simulink model "PMSM_STATE_SS_AR222"  (R2021a)
settings: Solver=ode45  StartTime=0.0  StopTime=2.5  RelTol=1e-3
values from neighbouring files (symbols this model uses):
  b = (Trt*R1)/(2*Tmu_i*ki*kdt)    [PMSM_DQ_Data3.m]
  b2 = (J1)/(2*Tmu_w*cm*kds)    (= 1.84257075472)    [PMSM_DQ_Data3.m]
  cm = 1.5*p*wf    (= 0.325632)    [PMSM_DQ_Data3.m]
  Imax = iqn    (= 21.9265919811)    [PMSM_DQ_Data3.m]
  J1 = 0.00048    [PMSM_DQ_Data3.m]
  kds = 1    [PMSM_DQ_Data3.m]
  kdt = 1    [PMSM_DQ_Data3.m]
  ki = Udc/5    [PMSM_DQ_Data3.m]
  Kml = 0.3266    [Parameters_for_Friction.m]
  Kv2 = 0    [Parameters_for_Friction.m]
  L1 = 0.001015    [PMSM_DQ_Data3.m]
  Mc = 0.0405    [Parameters_for_Friction.m]
  Ms = 0.0467    [Parameters_for_Friction.m]
  omega_2s = 10.47    [Parameters_for_Friction.m]
  p = 4    [PMSM_DQ_Data3.m]
  R1 = 0.24    [PMSM_DQ_Data3.m]
  ro_0 = 100    [Parameters_for_Friction.m]
  ro_1 = 0.923    [Parameters_for_Friction.m]
  T1 = L1/R1    (= 0.00422916666667)    [PMSM_DQ_Data3.m]
  Ti = 1/f_inv    (= 0.0002)    [PMSM_DQ_Data3.m]
  Tmin = 2e-4    (= 0.0002)    [Parameters_for_Friction.m]
  Trt = T1    (= 0.00422916666667)    [PMSM_DQ_Data3.m]
  Trt2 = 4*Tmu_w    (= 0.0016)    [PMSM_DQ_Data3.m]
  Umax = sqrt((p*wn*L1*iqn)^2+(En^2))    [PMSM_DQ_Data3.m]
  wf = 0.06784*0.8    (= 0.054272)    [PMSM_DQ_Data3.m]
settings Model: Creator=User  LastModifiedBy=dns
settings SolverCC: AlgebraicLoopSolver=TrustRegion
settings DataIOCC: LimitDataPoints=on  SaveFormat=Array  ReturnWorkspaceOutputs=off
settings OptimizationCC: BlockReduction=off  BooleanDataType=off  LifeSpan=inf
settings DebuggingCC: SaveWithParameterizedLinksMsg=none  UnderspecifiedInitializationDetection=Classic  MergeDetectMultiDrivingBlocksExec=none  SignalResolutionControl=TryResolveAllWithWarning  SFUnexpectedBacktrackingDiag=warning  SFNoUnconditionalDefaultTransitionDiag=warning  SFExecutionAtInitializationDiag=none  SFMachineParentedDataDiag=warning  ArithmeticOperatorsInVariantConditions=warning
settings HardwareCC: ProdBitPerPointer=32  ProdBitPerSizeT=32  ProdBitPerPtrDiffT=32  ProdLargestAtomicFloat=None  ProdIntDivRoundTo=Undefined  ProdEndianess=Unspecified  ProdWordSize=32  ProdHWDeviceType=32-bit Generic  TargetUnknown=on
settings ModelReferenceCC: PropagateSignalLabelsOutOfModel=off
settings SFSimCC: SimUseLocalCustomCode=off  CustomCodeUndefinedFunction=UseInterfaceOnly
settings RTWCC: RTWUseLocalCustomCode=off
settings CodeAppCC: StateflowObjectComments=on
settings GRTTargetCC: TargetLangStandard=C89/C90 (ANSI)
settings ConfigComp: CovMetricSettings=dw  CovSaveCumulativeToWorkspaceVar=on  CovSaveSingleToWorkspaceVar=on  CovExternalEMLEnable=off  CovSFcnEnable=off

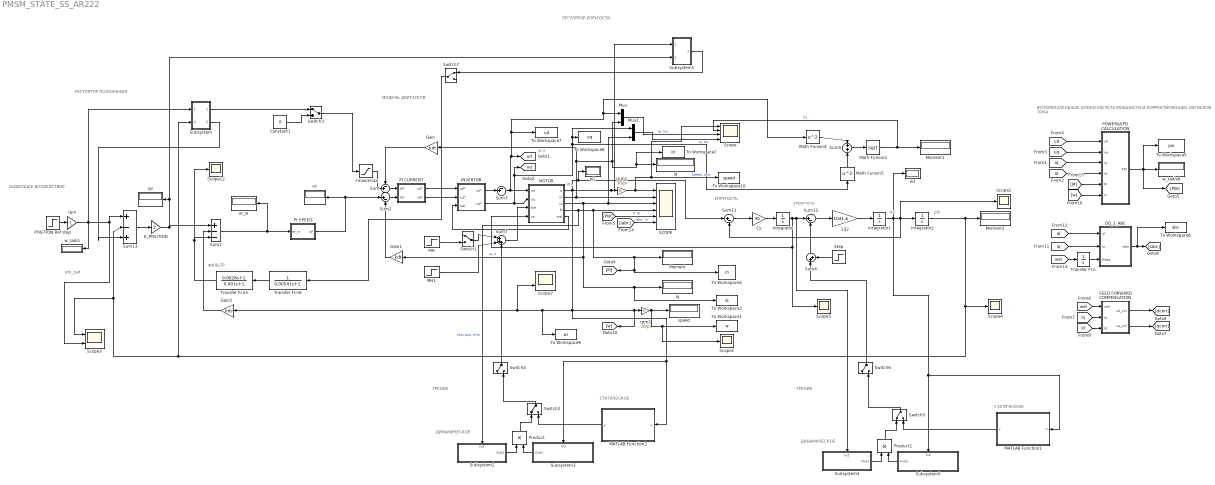
== system PMSM_STATE_SS_AR222 ==
  note: МОДЕЛЬ ДВИГАТЕЛЯ
  note: ФИЛЬТР
  note: ВСПОМОГАТЕЛЬНЫЕ БЛОКИ РАСЧЕТА МОЩНОСТИ
      | И КОРРЕКТИРУЮЩИХ СИГНАЛОВ ТОКА
  note: ДИНАМИЧЕСКОЕ
  note: СТАТИЧЕСКОЕ
  note: ТРЕНИЕ
  note: ТРЕНИЕ
  note: УПРУГОСТЬ
  note: РЕГУЛЯТОР УПРУГОСТИ
  note: РЕГУЛЯТОР ПОЛОЖЕНИЯ
  note: ЗАДАЮЩЕЕ ВОЗДЕЙСТВИЕ
  note: phi_zad
  note: упругость
  note: phi
  note: w2
  note: w1
  note: ДИНАМИЧЕСКОЕ
  note: СТАТИЧЕСКОЕ
  -Imax/Imax : Saturate  UpperLimit=Imax  LowerLimit=-Imax
  1/J2 : Gain  Gain=1041.6
  Constant1 : Constant  Value=0
  Cy : Gain  Gain=30
  DQ_2_ABC : Subsystem
  FEED FORWARD COMPENSATION : Subsystem
  Gain : Gain  Gain=kdt
  Gain1 : Gain  Gain=kdt
  Gain2 : Gain  Gain=kds
  INVERTOR : Subsystem
  Integrator : Integrator
  Integrator1 : Integrator
  Integrator2 : Integrator
  K_POSITION : Gain  Gain=3
  MATLAB Function1 : MATLAB Function  TreatAsAtomicUnit=on
  MATLAB Function2 : MATLAB Function  TreatAsAtomicUnit=on
  MH : Step  Time=0.15  After=3  SampleTime=0
  MH1 : Step  Time=0.2  After=0  SampleTime=0
  MOTOR : Subsystem
  Math Funion3 : Math  Operator=sqrt  SignedPower=on  SaturateOnIntegerOverflow=on
  Math Funion4 : Math  Operator=square  SignedPower=on  SaturateOnIntegerOverflow=on
  Math Funion5 : Math  Operator=square  SignedPower=on  SaturateOnIntegerOverflow=on
  Moment : Display
  Moment1 : Display
  Moment2 : Display
  Mux : Mux  Inputs=2
  Mux1 : Mux  Inputs=2
  PI CURRENT : Subsystem
  PI SPEED : Subsystem
  POSITION Ref step : Step  Time=0  After=0.1  SampleTime=0
  POWER&KPD CALCULATION : Subsystem
  Product : Product
  Product1 : Product
  SCOPE : Scope  NumInputPorts=6
  Scope : Scope  NumInputPorts=4
  Scope{1..2,4..5,12} (5 alike) : Scope
  Scope3 : Scope  NumInputPorts=2
  Scope7 : Scope  NumInputPorts=2
  Step : Step  After=0.105  SampleTime=0
  Subsystem : Subsystem
  Subsystem1 : Subsystem
  Subsystem2 : Subsystem
      settings: PortSchema="{\"entries\":[{\"content\":{\"sides\":[{\"content\":{\"connectorIds\":[]},\"type\":\"ConnectorPlacement.EquallySpacedRectSide\",\"uuid\":\"9e1ea793-1db2-4017-bc49-e2c095734c7f\"},{\"content\":{\"connectorIds\":[\"Out1\"],\"side\":\"RIGHT\"},\"type\":\"ConnectorPlacement.EquallySpacedRectSide\",\"uuid\":\"98a308e3-3e34-4e0b-b6ca-8e736cee5fdb\"},{\"content\":{\"connectorIds\":[\"In1\"],\"side\":\"TOP\"},\"type\":\"ConnectorPlacement.EquallySpacedRectSide\",\"uuid\":\"dcd5dfb1-aa8a-4a98-afa2-4364732e604f\"}]},\"type\":\"ConnectorPlacement.EquallySpacedConnector\",\"uuid\":\"fb12f03b-8158-4b93-b611-64d89b903ac2\"}],\"packageUris\":[\"http://schema.mathworks.com/mf0/Connector/R2020b\"],\"version\":\"1.0\"}"
      mask Display: image('Untitled2.png');
  Subsystem3 : Subsystem
      settings: PortSchema="{\"entries\":[{\"content\":{\"sides\":[{\"content\":{\"connectorIds\":[]},\"type\":\"ConnectorPlacement.EquallySpacedRectSide\",\"uuid\":\"9e1ea793-1db2-4017-bc49-e2c095734c7f\"},{\"content\":{\"connectorIds\":[\"Out1\"],\"side\":\"RIGHT\"},\"type\":\"ConnectorPlacement.EquallySpacedRectSide\",\"uuid\":\"98a308e3-3e34-4e0b-b6ca-8e736cee5fdb\"},{\"content\":{\"connectorIds\":[\"In1\"],\"side\":\"TOP\"},\"type\":\"ConnectorPlacement.EquallySpacedRectSide\",\"uuid\":\"dcd5dfb1-aa8a-4a98-afa2-4364732e604f\"}]},\"type\":\"ConnectorPlacement.EquallySpacedConnector\",\"uuid\":\"fb12f03b-8158-4b93-b611-64d89b903ac2\"}],\"packageUris\":[\"http://schema.mathworks.com/mf0/Connector/R2020b\"],\"version\":\"1.0\"}"
      mask Display: image('Untitled3.png');
  Subsystem4 : Subsystem
      settings: PortSchema="{\"entries\":[{\"content\":{\"sides\":[{\"content\":{\"connectorIds\":[]},\"type\":\"ConnectorPlacement.EquallySpacedRectSide\",\"uuid\":\"9e1ea793-1db2-4017-bc49-e2c095734c7f\"},{\"content\":{\"connectorIds\":[\"Out1\"],\"side\":\"RIGHT\"},\"type\":\"ConnectorPlacement.EquallySpacedRectSide\",\"uuid\":\"98a308e3-3e34-4e0b-b6ca-8e736cee5fdb\"},{\"content\":{\"connectorIds\":[\"In1\"],\"side\":\"TOP\"},\"type\":\"ConnectorPlacement.EquallySpacedRectSide\",\"uuid\":\"dcd5dfb1-aa8a-4a98-afa2-4364732e604f\"}]},\"type\":\"ConnectorPlacement.EquallySpacedConnector\",\"uuid\":\"fb12f03b-8158-4b93-b611-64d89b903ac2\"}],\"packageUris\":[\"http://schema.mathworks.com/mf0/Connector/R2020b\"],\"version\":\"1.0\"}"
      mask Display: image('Untitled2.png');
  Subsystem5 : Subsystem
      settings: PortSchema="{\"entries\":[{\"content\":{\"sides\":[{\"content\":{\"connectorIds\":[]},\"type\":\"ConnectorPlacement.EquallySpacedRectSide\",\"uuid\":\"9e1ea793-1db2-4017-bc49-e2c095734c7f\"},{\"content\":{\"connectorIds\":[\"Out1\"],\"side\":\"RIGHT\"},\"type\":\"ConnectorPlacement.EquallySpacedRectSide\",\"uuid\":\"98a308e3-3e34-4e0b-b6ca-8e736cee5fdb\"},{\"content\":{\"connectorIds\":[\"In1\"],\"side\":\"TOP\"},\"type\":\"ConnectorPlacement.EquallySpacedRectSide\",\"uuid\":\"dcd5dfb1-aa8a-4a98-afa2-4364732e604f\"}]},\"type\":\"ConnectorPlacement.EquallySpacedConnector\",\"uuid\":\"fb12f03b-8158-4b93-b611-64d89b903ac2\"}],\"packageUris\":[\"http://schema.mathworks.com/mf0/Connector/R2020b\"],\"version\":\"1.0\"}"
      mask Display: image('Untitled3.png');
  Sum : Sum  Inputs=-+|
  Sum1 : Sum  Inputs=|+-
  Sum11 : Sum  Inputs=|+-
  Sum12 : Sum  Inputs=|+-
  Sum13 : Sum  Inputs=|+-+
  Sum2 : Sum  Inputs=|+--
  Sum3 : Sum  Inputs=-+|
  Sum4 : Sum  Inputs=|++
  Sum5 : Sum
  Sum7 : Sum  Inputs=|+++
  Switch{1..7} (7 alike) : ManualSwitch
  To Workspace1 : ToWorkspace  VariableName=w  SampleTime=-1
  To Workspace10 : ToWorkspace  VariableName=speed  SampleTime=-1
  To Workspace2 : ToWorkspace  VariableName=id  SampleTime=-1
  To Workspace3 : ToWorkspace  VariableName=iq  SampleTime=-1
  To Workspace4 : ToWorkspace  VariableName=m  SampleTime=-1
  To Workspace5 : ToWorkspace  VariableName=pw  SampleTime=-1
  To Workspace6 : ToWorkspace  VariableName=abc  SampleTime=-1
  To Workspace7 : ToWorkspace  VariableName=ud  SampleTime=-1
  To Workspace8 : ToWorkspace  VariableName=uq  SampleTime=-1
  To Workspace9 : ToWorkspace  VariableName=wr  SampleTime=-1
  Transfer Fcn : TransferFcn  Denominator=[1 0]
  Transfer Fcn5 : TransferFcn  Numerator=[0.0028 1]  Denominator=[0.001 1]
  Transfer Fcn6 : TransferFcn  Numerator=[0 1]  Denominator=[0.00541 1]
  er_w : Display
  id : Display
  iq : Display
  rpm : Gain
  rpm1 : Gain  Gain=30/pi
  rpm2 : Gain  Gain=30/pi
  speed : Display
  uc : Display
  up : Display
  w1 : Display
  w2 : Display
  w_rad/s : Display
  w_rad/s6 : Display
  tag scope: ud=global, uq=global
  wires:
  MOTOR/5(wel) -> INVERTOR/3(wel)
  rpm/1 -> Subsystem/1(In1), Scope3/2, Sum13/1, w_rad/s/1
  Gain/1 -> Sum/1
  Sum/1 -> PI CURRENT/1(Id*)
  [id] -> POWER&KPD CALCULATION/4(id)
  [iq] -> POWER&KPD CALCULATION/3(iq)
  POWER&KPD CALCULATION/1(PW) -> w_rad/s6/1, [PW], To Workspace5/1
  [PW] -> SCOPE/5  "P, W"
  MH/1 -> Switch1/2
  [wel] -> FEED FORWARD COMPENSATION/1(wel)
  Gain1/1 -> Sum1/2
  [iabc] -> SCOPE/6  "iabc,  A"
  rpm1/1 -> Scope/1, To Workspace10/1, SCOPE/1  "Speed, rpm"
  MOTOR/2(id) -> Gain/1, Mux/2, To Workspace2/1, id/1, SCOPE/2  "id, A"
  MOTOR/3(iq) -> iq/1, To Workspace3/1, Gain1/1, Mux1/2, SCOPE/3  "iq, A"
  MOTOR/4(M) -> Subsystem2/1(In2), Moment/1, To Workspace4/1, [M], SCOPE/4  "Moment, N*m"
  [M] -> POWER&KPD CALCULATION/5(M)
  [wel] -> Transfer Fcn/1
  [w] -> POWER&KPD CALCULATION/6(w)
  rpm2/1 -> speed/1, Scope1/1, To Workspace1/1
  DQ_2_ABC/1(iabc) -> [iabc], To Workspace6/1
  Transfer Fcn/1 -> DQ_2_ABC/3(theta)
  [id] -> DQ_2_ABC/1(id)
  [iq] -> DQ_2_ABC/2(iq)
  [iq] -> FEED FORWARD COMPENSATION/2(Iq)
  [id] -> FEED FORWARD COMPENSATION/3(Id)
  [ud] -> POWER&KPD CALCULATION/1(ud)
  [uq] -> POWER&KPD CALCULATION/2(uq)
  Sum3/1 -> [ud], Math Funion4/1, Mux/1, To Workspace7/1, MOTOR/1(ud)
  INVERTOR/2(uq*.) -> [uq], Mux1/1, To Workspace8/1, Math Funion5/1, MOTOR/2(uq)
  FEED FORWARD COMPENSATION/1(ud_cor) -> [dcorr]
  FEED FORWARD COMPENSATION/2(uq_cor) -> [qcorr]
  INVERTOR/1(ud*.) -> Sum3/2
  PI CURRENT/1(ud*) -> INVERTOR/1(ud*)
  Math Funion5/1 -> Sum5/2
  Math Funion4/1 -> Sum5/1
  Sum5/1 -> Math Funion3/1
  Math Funion3/1 -> Scope/2, Moment1/1  "U1"
  Mux/1 -> Scope/3  "Id, Ud"
  Mux1/1 -> Scope/4  "Iq, Uq"
  MOTOR/1(w) -> w1/1, Sum11/1, Subsystem1/1(In1), rpm1/1, Subsystem3/1(In2), MATLAB Function2/1(u), rpm2/1, [w], Gain2/1, Scope7/2, To Workspace9/1
  Sum2/1 -> PI SPEED/1(er_w), er_w/1
  PI SPEED/1(iq*) -> uc/1, Sum1/1
  Constant1/1 -> Switch3/2
  Switch1/1 -> Sum7/1
  MH1/1 -> Sum7/2
  -Imax/Imax/1 -> Sum/2
  POSITION Ref step/1 -> rpm/1
  Sum11/1 -> Cy/1
  Cy/1 -> Integrator/1
  Sum12/1 -> 1/J2/1
  1/J2/1 -> Integrator1/1
  Integrator2/1 -> Scope4/1, Subsystem/2(In2), Sum13/2, Scope3/1, Moment2/1
  K_POSITION/1 -> Sum2/1, Subsystem1/2(In2), up/1
  Sum13/1 -> K_POSITION/1
  Switch3/1 -> -Imax/Imax/1
  Sum1/1 -> PI CURRENT/2(Iq*)
  PI CURRENT/2(uq*) -> INVERTOR/2(uq*)
  Gain2/1 -> Sum2/2
  Transfer Fcn5/1 -> Sum2/3, Scope12/1
  Transfer Fcn6/1 -> Transfer Fcn5/1
  Sum7/1 -> MOTOR/3(MH)
  Subsystem/1(Out1) -> Switch3/1
  Subsystem1/1(Out1) -> Switch7/1
  MATLAB Function2/1(y) -> Switch2/2
  Product/1 -> Switch2/1
  Subsystem3/1(Out1) -> Product/2
  Subsystem2/1(Out1) -> Product/1
  Switch2/1 -> Switch4/2
  Switch4/1 -> Sum7/3
  Product1/1 -> Switch5/1
  Integrator1/1 -> w2/1, Subsystem5/1(In2), MATLAB Function1/1(u), Scope2/1, Sum11/2, Integrator2/1
  MATLAB Function1/1(y) -> Switch5/2
  Subsystem4/1(Out1) -> Product1/1
  Subsystem5/1(Out1) -> Product1/2
  Integrator/1 -> Scope5/1, MOTOR/4(up), Subsystem4/1(In2), Sum12/1
  Switch5/1 -> Switch6/2
  Subsystem/2(Out2) -> Sum13/3
  Switch7/1 -> Transfer Fcn6/1
  Step/1 -> Sum4/2
  Switch6/1 -> Sum4/1
  Sum4/1 -> Sum12/2

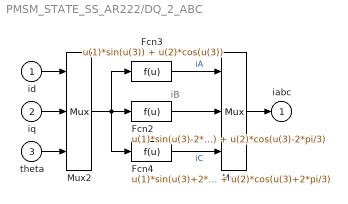
== system PMSM_STATE_SS_AR222/DQ_2_ABC ==
  note: iB
  id : Inport
  iq : Inport  Port=2
  theta : Inport  Port=3
  Fcn2 : Fcn  Expr=u(1)*sin(u(3)-2*pi/3) + u(2)*cos(u(3)-2*pi/3)
  Fcn3 : Fcn  Expr=u(1)*sin(u(3)) + u(2)*cos(u(3))
  Fcn4 : Fcn  Expr=u(1)*sin(u(3)+2*pi/3) + u(2)*cos(u(3)+2*pi/3)
  Mux2 : Mux  Inputs=3
  Mux3 : Mux  Inputs=3
  iabc : Outport  InitialOutput=0  VectorParamsAs1DForOutWhenUnconnected=off
  wires:
  id/1 -> Mux2/1
  iq/1 -> Mux2/2
  theta/1 -> Mux2/3
  Mux2/1 -> Fcn2/1, Fcn3/1, Fcn4/1
  Fcn3/1 -> Mux3/1  "iA"
  Fcn2/1 -> Mux3/2
  Fcn4/1 -> Mux3/3  "iC"
  Mux3/1 -> iabc/1

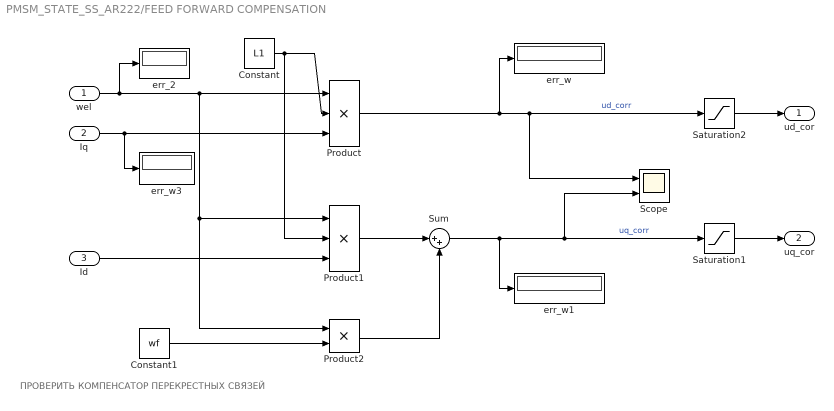
== system PMSM_STATE_SS_AR222/FEED FORWARD COMPENSATION ==
  note: ПРОВЕРИТЬ КОМПЕНСАТОР ПЕРЕКРЕСТНЫХ СВЯЗЕЙ
  wel : Inport
  Iq : Inport  Port=2
  Id : Inport  Port=3
  Constant : Constant  Value=L1
  Constant1 : Constant  Value=wf
  Product : Product  Inputs=3  RndMeth=Zero
  Product1 : Product  Inputs=3  RndMeth=Zero
  Product2 : Product  RndMeth=Zero
  Saturation1 : Saturate  UpperLimit=Umax  LowerLimit=-Umax
  Saturation2 : Saturate  UpperLimit=Umax  LowerLimit=-Umax
  Scope : Scope  NumInputPorts=2
  Sum : Sum  Inputs=|++
  err_2 : Display
  err_w : Display
  err_w1 : Display
  err_w3 : Display
  ud_cor : Outport  VectorParamsAs1DForOutWhenUnconnected=off
  uq_cor : Outport  Port=2  VectorParamsAs1DForOutWhenUnconnected=off
  wires:
  wel/1 -> err_2/1, Product/1, Product1/1, Product2/1
  Constant/1 -> Product/2, Product1/2
  Iq/1 -> Product/3, err_w3/1
  Product1/1 -> Sum/1
  Sum/1 -> err_w1/1, Scope/2, Saturation1/1  "uq_corr"
  Id/1 -> Product1/3
  Product2/1 -> Sum/2
  Constant1/1 -> Product2/2
  Product/1 -> err_w/1, Scope/1, Saturation2/1  "ud_corr"
  Saturation2/1 -> ud_cor/1
  Saturation1/1 -> uq_cor/1

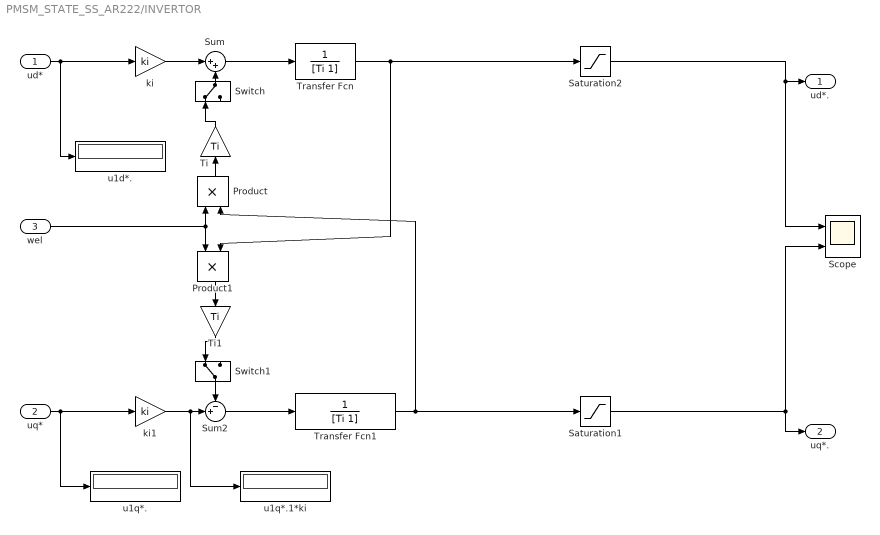
== system PMSM_STATE_SS_AR222/INVERTOR ==
  ud* : Inport
  uq* : Inport  Port=2
  wel : Inport  Port=3
  Product : Product  RndMeth=Zero
  Product1 : Product  RndMeth=Zero
  Saturation1 : Saturate  UpperLimit=Umax  LowerLimit=-Umax
  Saturation2 : Saturate  UpperLimit=Umax  LowerLimit=-Umax
  Scope : Scope  NumInputPorts=2
  Sum : Sum  Inputs=|++
  Sum2 : Sum  Inputs=-+|
  Switch : ManualSwitch
  Switch1 : ManualSwitch
  Ti : Gain  Gain=Ti
  Ti1 : Gain  Gain=Ti
  Transfer Fcn : TransferFcn  Denominator=[Ti 1]
  Transfer Fcn1 : TransferFcn  Denominator=[Ti 1]
  ki : Gain  Gain=ki
  ki1 : Gain  Gain=ki
  u1d*. : Display
  u1q*. : Display
  u1q*.1*ki : Display
  ud*. : Outport  VectorParamsAs1DForOutWhenUnconnected=off
  uq*. : Outport  Port=2  VectorParamsAs1DForOutWhenUnconnected=off
  wires:
  ud*/1 -> u1d*./1, ki/1
  ki/1 -> Sum/1
  Product/1 -> Ti/1
  Transfer Fcn/1 -> Product1/2, Saturation2/1
  uq*/1 -> u1q*./1, ki1/1
  Transfer Fcn1/1 -> Product/2, Saturation1/1
  Product1/1 -> Ti1/1
  ki1/1 -> Sum2/2, u1q*.1*ki/1
  Sum2/1 -> Transfer Fcn1/1
  wel/1 -> Product/1, Product1/1
  Ti/1 -> Switch/1
  Switch/1 -> Sum/2
  Ti1/1 -> Switch1/1
  Switch1/1 -> Sum2/1
  Sum/1 -> Transfer Fcn/1
  Saturation2/1 -> ud*./1, Scope/1
  Saturation1/1 -> uq*./1, Scope/2

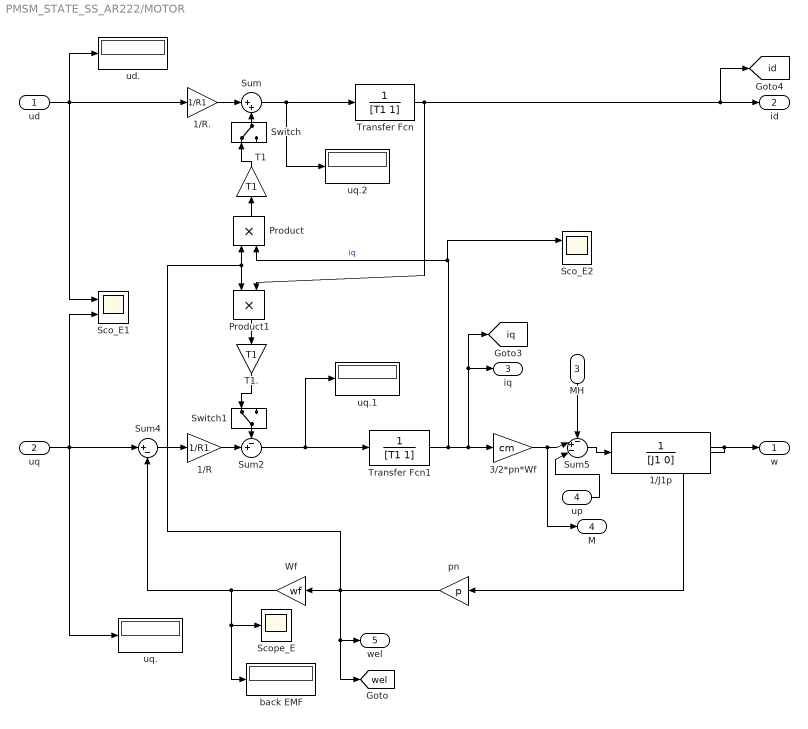
== system PMSM_STATE_SS_AR222/MOTOR ==
  ud : Inport
  uq : Inport  Port=2
  MH : Inport  Port=3
  up : Inport  Port=4
  1/J1p : TransferFcn  Denominator=[J1 0]
  1/R : Gain  Gain=1/R1
  1/R. : Gain  Gain=1/R1
  3/2*pn*Wf : Gain  Gain=cm
  Product : Product  RndMeth=Zero
  Product1 : Product  RndMeth=Zero
  Sco_E1 : Scope  NumInputPorts=2
  Sco_E2 : Scope  NumInputPorts=2
  Scope_E : Scope
  Sum : Sum  Inputs=|++
  Sum2 : Sum  Inputs=-+|
  Sum4 : Sum  Inputs=|+-
  Sum5 : Sum  Inputs=-+-|
  Switch : ManualSwitch
  Switch1 : ManualSwitch
  T1 : Gain  Gain=T1
  T1. : Gain  Gain=T1
  Transfer Fcn : TransferFcn  Denominator=[T1 1]
  Transfer Fcn1 : TransferFcn  Denominator=[T1 1]
  Wf : Gain  Gain=wf
  back EMF : Display
  pn : Gain  Gain=p
  ud. : Display
  uq. : Display
  uq.1 : Display
  uq.2 : Display
  w : Outport  VectorParamsAs1DForOutWhenUnconnected=off
  id : Outport  Port=2  VectorParamsAs1DForOutWhenUnconnected=off
  iq : Outport  Port=3  VectorParamsAs1DForOutWhenUnconnected=off
  M : Outport  Port=4  VectorParamsAs1DForOutWhenUnconnected=off
  wel : Outport  Port=5  VectorParamsAs1DForOutWhenUnconnected=off
  tag scope: id=global, iq=global, wel=global
  wires:
  ud/1 -> ud./1, 1/R./1, Sco_E1/1
  1/R./1 -> Sum/1
  Product/1 -> T1/1
  Sum/1 -> Transfer Fcn/1, uq.2/1
  Transfer Fcn/1 -> Product1/2, id/1, [id]
  Transfer Fcn1/1 -> Sco_E2/1, Product/2, 3/2*pn*Wf/1, iq/1, [iq]  "iq"
  Product1/1 -> T1./1
  1/R/1 -> Sum2/2
  Sum2/1 -> Transfer Fcn1/1, uq.1/1
  Sum4/1 -> 1/R/1
  Wf/1 -> back EMF/1, Scope_E/1, Sum4/2
  pn/1 -> Wf/1, wel/1, [wel], Product/1, Product1/1
  MH/1 -> Sum5/1
  Sum5/1 -> 1/J1p/1
  1/J1p/1 -> pn/1, w/1
  3/2*pn*Wf/1 -> M/1, Sum5/2
  uq/1 -> uq./1, Sum4/1, Sco_E1/2
  T1/1 -> Switch/1
  Switch/1 -> Sum/2
  Switch1/1 -> Sum2/1
  T1./1 -> Switch1/1
  up/1 -> Sum5/3

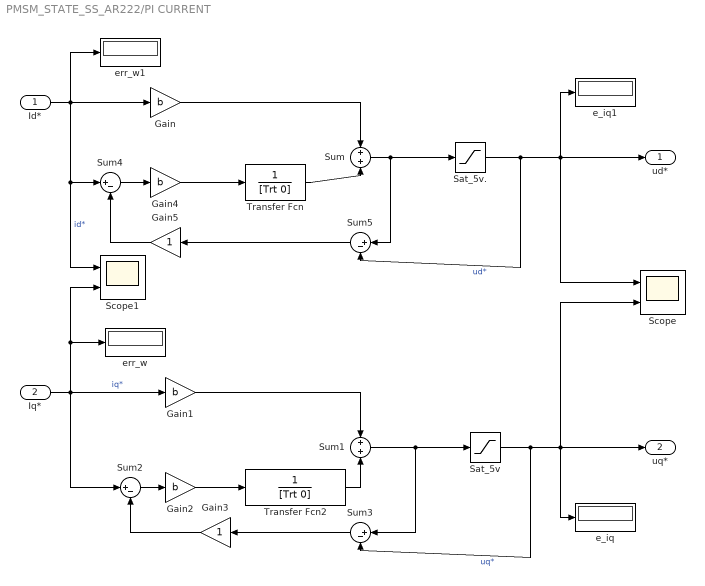
== system PMSM_STATE_SS_AR222/PI CURRENT ==
  Id* : Inport
  Iq* : Inport  Port=2
  Gain{,1..2,4} (4 alike) : Gain  Gain=b
  Gain3 : Gain
  Gain5 : Gain
  Sat_5v : Saturate  UpperLimit=5  LowerLimit=-5
  Sat_5v. : Saturate  UpperLimit=5  LowerLimit=-5
  Scope : Scope  NumInputPorts=2
  Scope1 : Scope  NumInputPorts=2
  Sum : Sum
  Sum1 : Sum
  Sum{2..5} (4 alike) : Sum  Inputs=|+-
  Transfer Fcn : TransferFcn  Denominator=[Trt 0]
  Transfer Fcn2 : TransferFcn  Denominator=[Trt 0]
  e_iq : Display
  e_iq1 : Display
  err_w : Display
  err_w1 : Display
  ud* : Outport  VectorParamsAs1DForOutWhenUnconnected=off
  uq* : Outport  Port=2  VectorParamsAs1DForOutWhenUnconnected=off
  wires:
  Gain1/1 -> Sum1/1
  Iq*/1 -> err_w/1, Scope1/2, Gain1/1, Sum2/1  "iq*"
  Sum1/1 -> Sum3/1, Sat_5v/1
  Sat_5v/1 -> Sum3/2, Scope/2, uq*/1, e_iq/1  "uq*"
  Sum3/1 -> Gain3/1
  Sum2/1 -> Gain2/1
  Gain2/1 -> Transfer Fcn2/1
  Gain3/1 -> Sum2/2
  Id*/1 -> Gain/1, err_w1/1, Sum4/1, Scope1/1  "id*"
  Sum/1 -> Sum5/1, Sat_5v./1
  Gain/1 -> Sum/1
  Gain4/1 -> Transfer Fcn/1
  Sum4/1 -> Gain4/1
  Gain5/1 -> Sum4/2
  Sum5/1 -> Gain5/1
  Sat_5v./1 -> Sum5/2, e_iq1/1, Scope/1, ud*/1  "ud*"
  Transfer Fcn/1 -> Sum/2
  Transfer Fcn2/1 -> Sum1/2

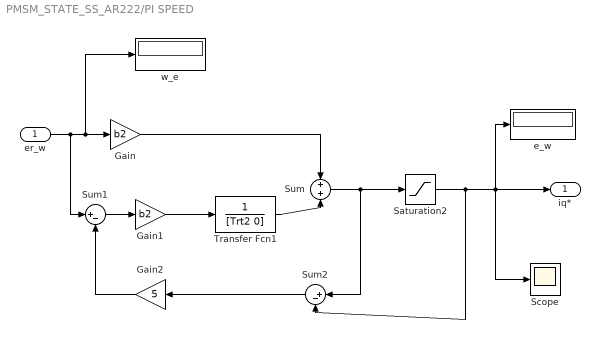
== system PMSM_STATE_SS_AR222/PI SPEED ==
  er_w : Inport
  Gain : Gain  Gain=b2
  Gain1 : Gain  Gain=b2
  Gain2 : Gain  Gain=5
  Saturation2 : Saturate  UpperLimit=Imax  LowerLimit=-Imax
  Scope : Scope
  Sum : Sum
  Sum1 : Sum  Inputs=|+-
  Sum2 : Sum  Inputs=|+-
  Transfer Fcn1 : TransferFcn  Denominator=[Trt2 0]
  e_w : Display
  w_e : Display
  iq* : Outport  VectorParamsAs1DForOutWhenUnconnected=off
  wires:
  Gain/1 -> Sum/1
  er_w/1 -> Gain/1, w_e/1, Sum1/1
  Sum/1 -> Saturation2/1, Sum2/1
  Saturation2/1 -> Sum2/2, iq*/1, Scope/1, e_w/1
  Gain1/1 -> Transfer Fcn1/1
  Sum1/1 -> Gain1/1
  Sum2/1 -> Gain2/1
  Gain2/1 -> Sum1/2
  Transfer Fcn1/1 -> Sum/2

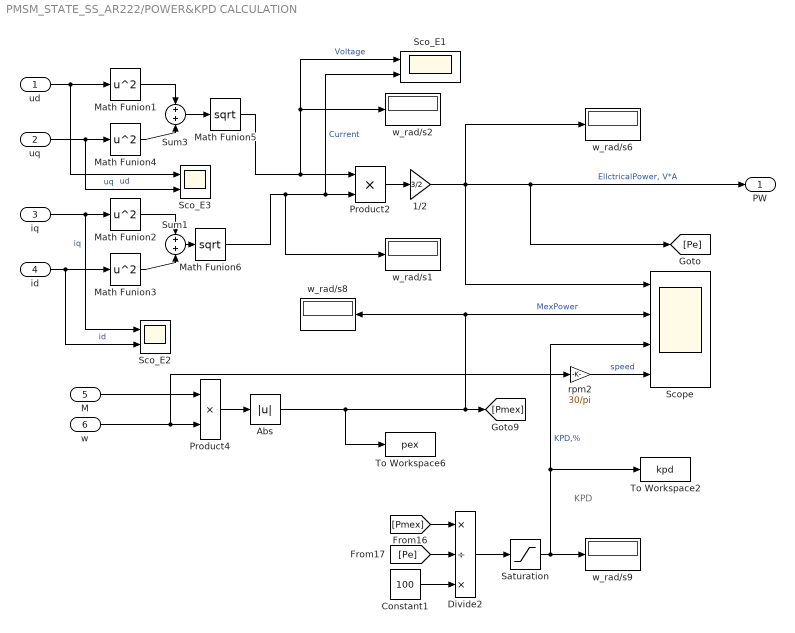
== system PMSM_STATE_SS_AR222/POWER&KPD CALCULATION ==
  note: KPD
  ud : Inport
  uq : Inport  Port=2
  iq : Inport  Port=3
  id : Inport  Port=4
  M : Inport  Port=5
  w : Inport  Port=6
  1/2 : Gain  Gain=3/2
  Abs : Abs
  Constant1 : Constant  Value=100
  Divide2 : Product  Inputs=*/*
  Math Funion{1..4} (4 alike) : Math  Operator=square  SignedPower=on  SaturateOnIntegerOverflow=on
  Math Funion5 : Math  Operator=sqrt  SignedPower=on  SaturateOnIntegerOverflow=on
  Math Funion6 : Math  Operator=sqrt  SignedPower=on  SaturateOnIntegerOverflow=on
  Product2 : Product  RndMeth=Zero
  Product4 : Product  RndMeth=Zero
  Saturation : Saturate  UpperLimit=100  LowerLimit=0
  Sco_E1 : Scope  NumInputPorts=2
  Sco_E2 : Scope  NumInputPorts=2
  Sco_E3 : Scope  NumInputPorts=2
  Scope : Scope  NumInputPorts=4
  Sum1 : Sum
  Sum3 : Sum
  To Workspace2 : ToWorkspace  VariableName=kpd  SampleTime=-1
  To Workspace6 : ToWorkspace  VariableName=pex  SampleTime=-1
  rpm2 : Gain  Gain=30/pi
  w_rad/s{1..2,6,8..9} (5 alike) : Display
  PW : Outport  VectorParamsAs1DForOutWhenUnconnected=off
  wires:
  Product4/1 -> Abs/1
  M/1 -> Product4/1
  w/1 -> Product4/2, rpm2/1
  Constant1/1 -> Divide2/3
  Divide2/1 -> Saturation/1
  [Pmex] -> Divide2/1
  [Pe] -> Divide2/2
  Saturation/1 -> w_rad/s9/1, Scope/3, To Workspace2/1  "KPD,%"
  Math Funion2/1 -> Sum1/1
  Math Funion3/1 -> Sum1/2
  Math Funion4/1 -> Sum3/2
  Math Funion1/1 -> Sum3/1
  Sum3/1 -> Math Funion5/1
  Sum1/1 -> Math Funion6/1
  Math Funion5/1 -> Product2/1, Sco_E1/1, w_rad/s2/1  "Voltage"
  Product2/1 -> 1/2/1
  ud/1 -> Math Funion1/1, Sco_E3/1  "ud"
  uq/1 -> Math Funion4/1, Sco_E3/2  "uq"
  iq/1 -> Math Funion2/1, Sco_E2/1  "iq"
  id/1 -> Sco_E2/2, Math Funion3/1  "id"
  1/2/1 -> w_rad/s6/1, Scope/1, [Pe], PW/1  "EllctricalPower, V*A"
  Abs/1 -> [Pmex], Scope/2, w_rad/s8/1, To Workspace6/1  "MexPower"
  Math Funion6/1 -> Product2/2, Sco_E1/2, w_rad/s1/1  "Current"
  rpm2/1 -> Scope/4  "speed"

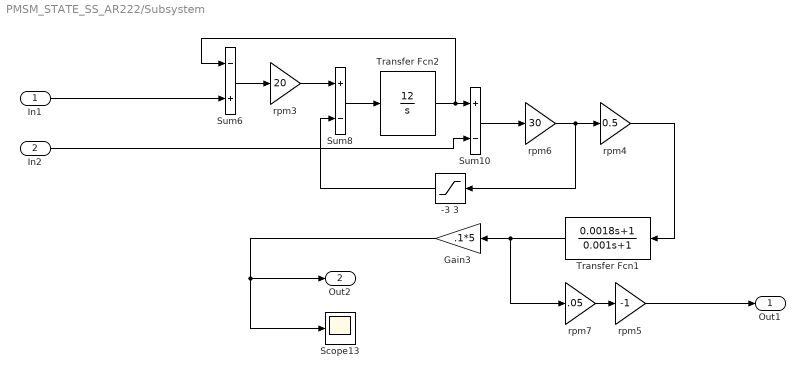
== system PMSM_STATE_SS_AR222/Subsystem ==
  In1 : Inport
  In2 : Inport  Port=2
  -3 3 : Saturate  UpperLimit=3  LowerLimit=-3
  Gain3 : Gain  Gain=.1*5
  Scope13 : Scope
  Sum10 : Sum  Inputs=+-
  Sum6 : Sum  Inputs=-+
  Sum8 : Sum  Inputs=+-
  Transfer Fcn1 : TransferFcn  Numerator=[0.0018 1]  Denominator=[0.001 1]
  Transfer Fcn2 : TransferFcn  Numerator=[12]  Denominator=[1 0]
  rpm3 : Gain  Gain=20
  rpm4 : Gain  Gain=0.5
  rpm5 : Gain  Gain=-1
  rpm6 : Gain  Gain=30
  rpm7 : Gain  Gain=.05
  Out1 : Outport
  Out2 : Outport  Port=2
  wires:
  rpm7/1 -> rpm5/1
  Transfer Fcn1/1 -> rpm7/1, Gain3/1
  Sum6/1 -> rpm3/1
  Gain3/1 -> Scope13/1, Out2/1
  rpm3/1 -> Sum8/1
  -3 3/1 -> Sum8/2
  Sum10/1 -> rpm6/1
  Sum8/1 -> Transfer Fcn2/1
  rpm6/1 -> rpm4/1, -3 3/1
  rpm4/1 -> Transfer Fcn1/1
  Transfer Fcn2/1 -> Sum6/1, Sum10/1
  In1/1 -> Sum6/2
  In2/1 -> Sum10/2
  rpm5/1 -> Out1/1

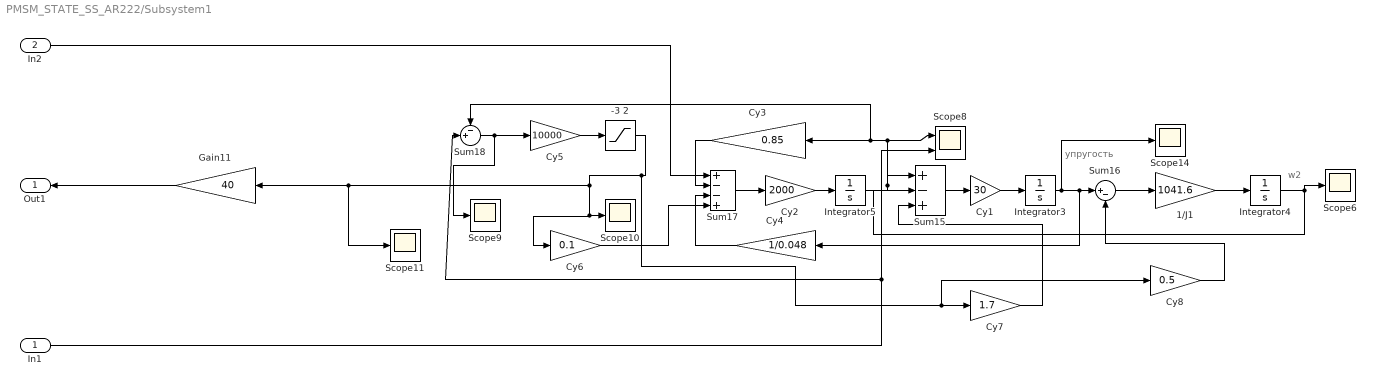
== system PMSM_STATE_SS_AR222/Subsystem1 ==
  note: упругость
  note: w2
  In1 : Inport
  In2 : Inport  Port=2
  -3 2 : Saturate  UpperLimit=0.5*2  LowerLimit=-0.5*2
  1/J1 : Gain  Gain=1041.6
  Cy1 : Gain  Gain=30
  Cy2 : Gain  Gain=2000
  Cy3 : Gain  Gain=0.85
  Cy4 : Gain  Gain=1/0.048
  Cy5 : Gain  Gain=10000
  Cy6 : Gain  Gain=0.1
  Cy7 : Gain  Gain=1.7
  Cy8 : Gain  Gain=0.5
  Gain11 : Gain  Gain=40
  Integrator3 : Integrator
  Integrator4 : Integrator
  Integrator5 : Integrator
  Scope{6,9..11,14} (5 alike) : Scope
  Scope8 : Scope  NumInputPorts=2
  Sum15 : Sum  Inputs=|+-+
  Sum16 : Sum  Inputs=|+-
  Sum17 : Sum  Inputs=+--+
  Sum18 : Sum  Inputs=-+|
  Out1 : Outport
  wires:
  Integrator5/1 -> Sum18/1, Cy3/1, Scope8/1, Sum15/1
  Cy7/1 -> Sum15/3
  In1/1 -> Scope8/2, Sum18/2
  Cy3/1 -> Sum17/2
  1/J1/1 -> Integrator4/1
  Cy6/1 -> Sum17/4
  Integrator3/1 -> Cy4/1, Sum16/1, Scope14/1
  Sum15/1 -> Cy1/1
  Sum18/1 -> Cy5/1, Scope9/1
  Integrator4/1 -> Scope6/1, Sum15/2
  Sum17/1 -> Cy2/1
  Cy4/1 -> Sum17/3
  Cy5/1 -> -3 2/1
  Cy2/1 -> Integrator5/1
  -3 2/1 -> Cy8/1, Cy7/1, Scope11/1, Gain11/1, Cy6/1, Scope10/1
  Cy1/1 -> Integrator3/1
  Cy8/1 -> Sum16/2
  Sum16/1 -> 1/J1/1
  Gain11/1 -> Out1/1
  In2/1 -> Sum17/1

== system PMSM_STATE_SS_AR222/Subsystem2 ==
  In2 : Inport
  Abs : Abs
  Add : Sum
  Constant1 : Constant
  Constant3 : Constant  Value=Kml
  Product : Product
  Scope1 : Scope
  Out1 : Outport  VectorParamsAs1DForOutWhenUnconnected=off
  wires:
  Constant3/1 -> Product/2
  Abs/1 -> Product/1
  Add/1 -> Out1/1, Scope1/1
  In2/1 -> Abs/1
  Product/1 -> Add/2
  Constant1/1 -> Add/1

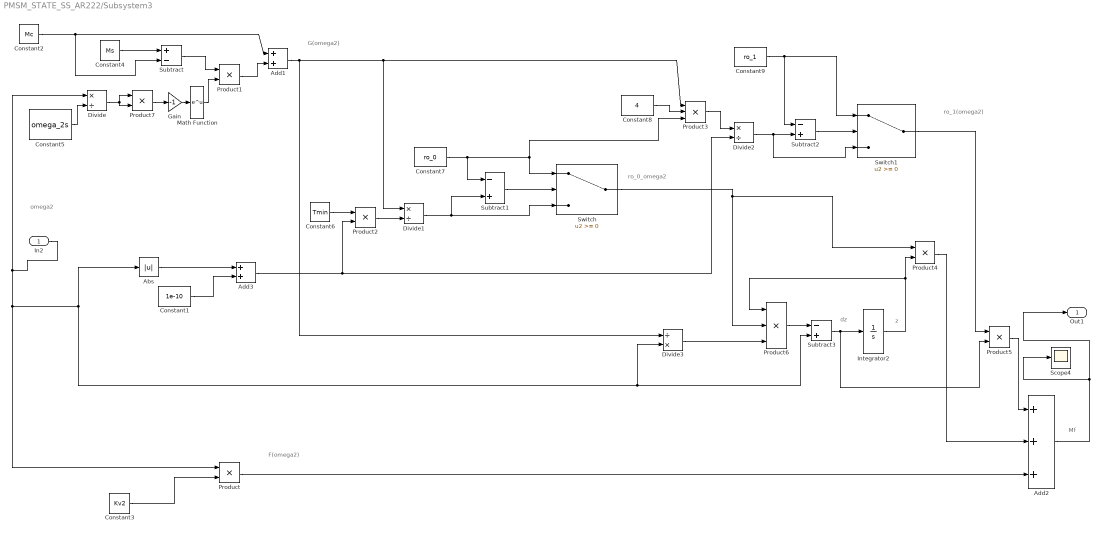
== system PMSM_STATE_SS_AR222/Subsystem3 ==
  note: Mf
  note: ro_0_omega2
  note: dz
  note: z
  note: G(omega2)
  note: ro_1(omega2)
  note: F(omega2)
  note: omega2
  In2 : Inport
  Abs : Abs
  Add1 : Sum
  Add2 : Sum  Inputs=+++
  Add3 : Sum
  Constant1 : Constant  Value=1e-10
  Constant2 : Constant  Value=Mc
  Constant3 : Constant  Value=Kv2
  Constant4 : Constant  Value=Ms
  Constant5 : Constant  Value=omega_2s
  Constant6 : Constant  Value=Tmin
  Constant7 : Constant  Value=ro_0
  Constant8 : Constant  Value=4
  Constant9 : Constant  Value=ro_1
  Divide : Product  Inputs=*/
  Divide1 : Product  Inputs=*/
  Divide2 : Product  Inputs=*/
  Divide3 : Product  Inputs=/*
  Gain : Gain  Gain=-1
  Integrator2 : Integrator
  Math Function : Math  SignedPower=on  SaturateOnIntegerOverflow=on
  Product{,1..2,4..5,7} (6 alike) : Product
  Product3 : Product  Inputs=3
  Product6 : Product  Inputs=3
  Scope4 : Scope
  Subtract : Sum  Inputs=+-
  Subtract1 : Sum  Inputs=-+
  Subtract2 : Sum  Inputs=-+
  Subtract3 : Sum  Inputs=-+
  Switch : Switch
  Switch1 : Switch
  Out1 : Outport  VectorParamsAs1DForOutWhenUnconnected=off
  wires:
  Constant1/1 -> Add3/2
  Constant3/1 -> Product/2
  Constant2/1 -> Subtract/2, Add1/1
  Constant4/1 -> Subtract/1
  Constant5/1 -> Divide/2
  Gain/1 -> Math Function/1
  Math Function/1 -> Product1/2
  Subtract/1 -> Product1/1
  Product1/1 -> Add1/2
  Abs/1 -> Add3/1
  Product2/1 -> Divide1/2
  Constant7/1 -> Product3/3, Switch/1, Subtract1/1
  Divide1/1 -> Switch/3, Subtract1/2
  Subtract1/1 -> Switch/2
  Add1/1 -> Divide3/1, Divide1/1, Product3/1
  Product3/1 -> Divide2/1
  Divide2/1 -> Switch1/3, Subtract2/2
  Constant9/1 -> Subtract2/1, Switch1/1
  Subtract2/1 -> Switch1/2
  Switch/1 -> Product6/2, Product4/1
  Subtract3/1 -> Product5/2, Integrator2/1
  Switch1/1 -> Product5/1
  Product6/1 -> Subtract3/1
  Integrator2/1 -> Product6/1, Product4/2
  Divide3/1 -> Product6/3
  Product5/1 -> Add2/1
  Product4/1 -> Add2/2
  Product/1 -> Add2/3
  Add2/1 -> Scope4/1, Out1/1
  In2/1 -> Abs/1, Divide3/2, Subtract3/2, Product/1, Divide/1
  Constant6/1 -> Product2/1
  Constant8/1 -> Product3/2
  Product7/1 -> Gain/1
  Divide/1 -> Product7/2, Product7/1
  Add3/1 -> Product2/2, Divide2/2

== system PMSM_STATE_SS_AR222/Subsystem4 ==
  In2 : Inport
  Abs : Abs
  Add : Sum
  Constant1 : Constant
  Constant3 : Constant  Value=Kml
  Product : Product
  Scope1 : Scope
  Out1 : Outport  VectorParamsAs1DForOutWhenUnconnected=off
  wires:
  Constant3/1 -> Product/2
  Abs/1 -> Product/1
  Add/1 -> Out1/1, Scope1/1
  In2/1 -> Abs/1
  Product/1 -> Add/2
  Constant1/1 -> Add/1

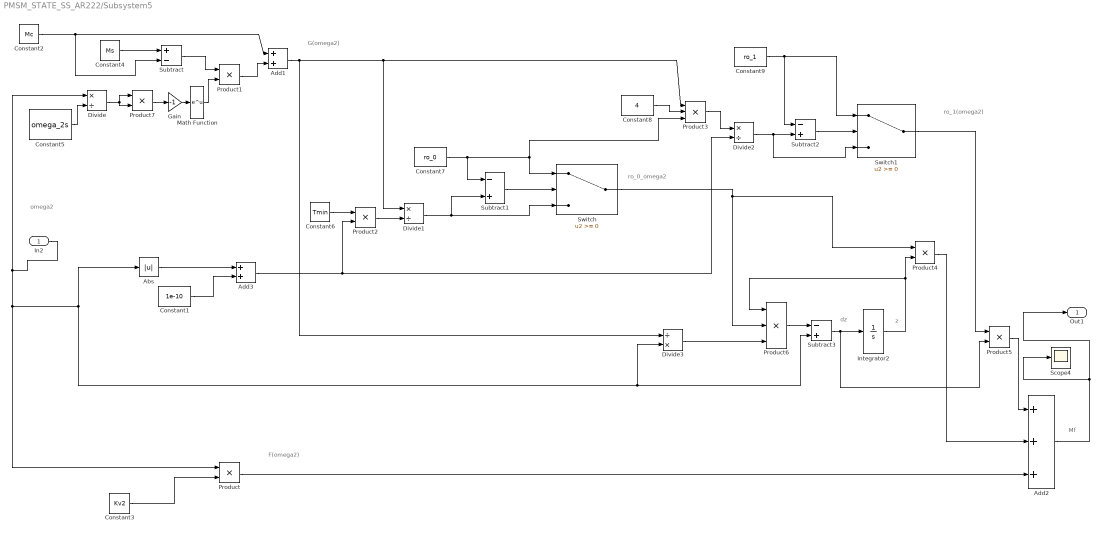
== system PMSM_STATE_SS_AR222/Subsystem5 ==
  note: Mf
  note: ro_0_omega2
  note: dz
  note: z
  note: G(omega2)
  note: ro_1(omega2)
  note: F(omega2)
  note: omega2
  In2 : Inport
  Abs : Abs
  Add1 : Sum
  Add2 : Sum  Inputs=+++
  Add3 : Sum
  Constant1 : Constant  Value=1e-10
  Constant2 : Constant  Value=Mc
  Constant3 : Constant  Value=Kv2
  Constant4 : Constant  Value=Ms
  Constant5 : Constant  Value=omega_2s
  Constant6 : Constant  Value=Tmin
  Constant7 : Constant  Value=ro_0
  Constant8 : Constant  Value=4
  Constant9 : Constant  Value=ro_1
  Divide : Product  Inputs=*/
  Divide1 : Product  Inputs=*/
  Divide2 : Product  Inputs=*/
  Divide3 : Product  Inputs=/*
  Gain : Gain  Gain=-1
  Integrator2 : Integrator
  Math Function : Math  SignedPower=on  SaturateOnIntegerOverflow=on
  Product{,1..2,4..5,7} (6 alike) : Product
  Product3 : Product  Inputs=3
  Product6 : Product  Inputs=3
  Scope4 : Scope
  Subtract : Sum  Inputs=+-
  Subtract1 : Sum  Inputs=-+
  Subtract2 : Sum  Inputs=-+
  Subtract3 : Sum  Inputs=-+
  Switch : Switch
  Switch1 : Switch
  Out1 : Outport  VectorParamsAs1DForOutWhenUnconnected=off
  wires:
  Constant1/1 -> Add3/2
  Constant3/1 -> Product/2
  Constant2/1 -> Subtract/2, Add1/1
  Constant4/1 -> Subtract/1
  Constant5/1 -> Divide/2
  Gain/1 -> Math Function/1
  Math Function/1 -> Product1/2
  Subtract/1 -> Product1/1
  Product1/1 -> Add1/2
  Abs/1 -> Add3/1
  Product2/1 -> Divide1/2
  Constant7/1 -> Product3/3, Switch/1, Subtract1/1
  Divide1/1 -> Switch/3, Subtract1/2
  Subtract1/1 -> Switch/2
  Add1/1 -> Divide3/1, Divide1/1, Product3/1
  Product3/1 -> Divide2/1
  Divide2/1 -> Switch1/3, Subtract2/2
  Constant9/1 -> Subtract2/1, Switch1/1
  Subtract2/1 -> Switch1/2
  Switch/1 -> Product6/2, Product4/1
  Subtract3/1 -> Product5/2, Integrator2/1
  Switch1/1 -> Product5/1
  Product6/1 -> Subtract3/1
  Integrator2/1 -> Product6/1, Product4/2
  Divide3/1 -> Product6/3
  Product5/1 -> Add2/1
  Product4/1 -> Add2/2
  Product/1 -> Add2/3
  Add2/1 -> Scope4/1, Out1/1
  In2/1 -> Abs/1, Divide3/2, Subtract3/2, Product/1, Divide/1
  Constant6/1 -> Product2/1
  Constant8/1 -> Product3/2
  Product7/1 -> Gain/1
  Divide/1 -> Product7/2, Product7/1
  Add3/1 -> Product2/2, Divide2/2

== matlab function PMSM_STATE_SS_AR222/MATLAB Function2 ==
  data: u input; y output
function y = fcn(u)
Mc=0.405;
Ms=0.465;
teta_omega2=1e-4;
% % % 
u_abs=abs(u);
u1=u_abs-teta_omega2;
if u_abs < teta_omega2
    y=u*Ms/teta_omega2;
else
    y1=-(abs(u_abs-teta_omega2));
    y2=exp(y1)*(Ms-Mc)+Mc;
    y=y2*sign(u);
end

== matlab function PMSM_STATE_SS_AR222/MATLAB Function1 ==
  data: u input; y output
function y = fcn(u)
Mc=0.405;
Ms=0.465;
teta_omega2=1e-4;
% % % 
u_abs=abs(u);
u1=u_abs-teta_omega2;
if u_abs < teta_omega2
    y=u*Ms/teta_omega2;
else
    y1=-(abs(u_abs-teta_omega2));
    y2=exp(y1)*(Ms-Mc)+Mc;
    y=y2*sign(u);
end
